simulink model "BetaMacs"  (R2023a)
settings: Solver=ode4  StartTime=0.0  StopTime=tsim  FixedStep=baseRate  RelTol=1e-6  AbsTol=1e-6
undefined symbols (not defined in the file): a1, a2, a3, b0, b1, b2, b3, baseRate, DiscIntNeverNeededParam, drop_states_ARM, drop_states_BLACK, drop_states_BLUE, drop_states_RED, F_Black_X_nominal, F_Black_Y_nominal, F_Blue_X_nominal, F_Blue_Y_nominal, F_red_X_nominal, F_red_Y_nominal, F_thrusters_BLACK, F_thrusters_BLUE, F_thrusters_RED, Gamma1_el, Gamma1_sh, Gamma1_wr, Gamma2_el, Gamma2_sh, Gamma2_wr, Gamma3_el, Gamma3_sh, Gamma3_wr, Gamma4_el, Gamma4_sh, Gamma4_wr, Gamma5_el, Gamma5_sh, Gamma5_wr, Gamma6_el, Gamma6_sh, Gamma6_wr, home_states_BLACK, home_states_BLUE, home_states_RED, IBLACK, IBLUE, IDIST, IEE, init_states_BLACK, init_states_BLUE, init_states_RED, IPROX, IRED, Kd_elarm, Kd_sharm, Kd_tb, Kd_tblue, Kd_tr, Kd_wrarm, Kd_xb, Kd_xblue ... (+48)
libraries: nvidiaSharedBlocks x9, MainLibrary x4, dspsigops x4, simulink x1
(part 2 of 11)

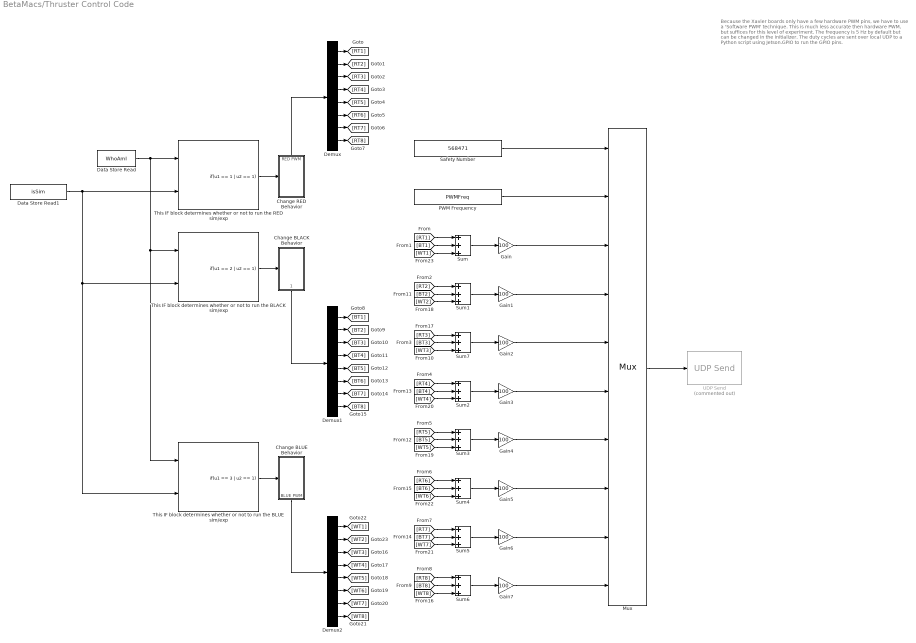
== system BetaMacs/Thruster Control Code ==
  note: Because the Xavier boards only have a few hardware PWM pins, we have to use a 'Software PWM' technique. This is much less accurate then hardware PWM, but suffices for this level of experiment.
      |
      | The frequency is 5 Hz by default but can be changed in the initializer. The duty cycles are sent over local UDP to a Python script using Jetson.GPIO to run the GPIO pins.
  Change BLACK Behavior : Subsystem  TreatAsAtomicUnit=on
  Change BLUE Behavior : Subsystem  TreatAsAtomicUnit=on
  Change RED Behavior : Subsystem  TreatAsAtomicUnit=on
  Data Store Read : DataStoreRead  DataStoreName=WhoAmI  IndexOptions=Index vector (dialog)  Indices=1  OutputSizes=1
  Data Store Read1 : DataStoreRead  DataStoreName=isSim  IndexOptions=Index vector (dialog)  Indices=1  OutputSizes=1
  Demux : Demux  Outputs=8
  Demux1 : Demux  Outputs=8
  Demux2 : Demux  Outputs=8
  Gain{,1..7} (8 alike) : Gain  Gain=100
  Mux : Mux  Inputs=10
  PWM Frequency : Constant  Value=PWMFreq
  Safety Number : Constant  Value=568471
  Sum{,1..7} (8 alike) : Sum  Inputs=+++
  This IF block determines whether or not to run the BLACK sim/exp : If  NumInputs=2  IfExpression=u1 == 2 | u2 == 1  ShowElse=off
  This IF block determines whether or not to run the BLUE sim/exp : If  NumInputs=2  IfExpression=u1 == 3 | u2 == 1  ShowElse=off
  "This IF block determines whether or not to run the RED sim/exp " : If  NumInputs=2  IfExpression=u1 == 1 | u2 == 1  ShowElse=off
  UDP Send : nvidiaSharedBlocks/UDP Send  Commented=on  remoteURL='127.0.0.1'  remotePort=48291  localURL='0.0.0.0'  localPortSource=Automatically determine  localPort=-1  sampletime=-1  blockPlatform=NVIDIA  separateLengthPort=0
      settings: LibrarySourceBlock=nvidiaNetworklib/UDP Send
  wires:
  Data Store Read1/1 -> This IF block determines whether or not to run the BLACK sim/exp/2, This IF block determines whether or not to run the BLUE sim/exp/2, "This IF block determines whether or not to run the RED sim/exp "/2
  "This IF block determines whether or not to run the RED sim/exp "/1 -> Change RED Behavior/Action
  This IF block determines whether or not to run the BLACK sim/exp/1 -> Change BLACK Behavior/Action
  Change RED Behavior/1(RED PWM) -> Demux/1
  Demux/1 -> [RT1]
  Demux/2 -> [RT2]
  Demux/3 -> [RT3]
  Demux/4 -> [RT4]
  Demux/5 -> [RT5]
  Demux/6 -> [RT6]
  Demux/7 -> [RT7]
  Demux/8 -> [RT8]
  Demux1/5 -> [BT5]
  Demux1/4 -> [BT4]
  Demux1/1 -> [BT1]
  Demux1/8 -> [BT8]
  Demux1/2 -> [BT2]
  Demux1/7 -> [BT7]
  Demux1/6 -> [BT6]
  Demux1/3 -> [BT3]
  Change BLACK Behavior/1(BLACK PWM) -> Demux1/1
  [RT1] -> Sum/1
  [BT1] -> Sum/2
  [RT2] -> Sum1/1
  [RT4] -> Sum2/1
  [RT5] -> Sum3/1
  [RT6] -> Sum4/1
  [RT7] -> Sum5/1
  [RT8] -> Sum6/1
  [BT8] -> Sum6/2
  [BT2] -> Sum1/2
  [BT5] -> Sum3/2
  [BT4] -> Sum2/2
  [BT7] -> Sum5/2
  [BT6] -> Sum4/2
  Sum/1 -> Gain/1
  Sum1/1 -> Gain1/1
  Data Store Read/1 -> This IF block determines whether or not to run the BLUE sim/exp/1, This IF block determines whether or not to run the BLACK sim/exp/1, "This IF block determines whether or not to run the RED sim/exp "/1
  This IF block determines whether or not to run the BLUE sim/exp/1 -> Change BLUE Behavior/Action
  Demux2/5 -> [WT5]
  Demux2/8 -> [WT8]
  Demux2/7 -> [WT7]
  Demux2/2 -> [WT2]
  Change BLUE Behavior/1(BLUE PWM) -> Demux2/1
  Demux2/1 -> [WT1]
  Demux2/4 -> [WT4]
  Demux2/3 -> [WT3]
  Demux2/6 -> [WT6]
  [WT8] -> Sum6/3
  [WT2] -> Sum1/3
  [WT5] -> Sum3/3
  [WT4] -> Sum2/3
  [WT7] -> Sum5/3
  [WT6] -> Sum4/3
  [WT1] -> Sum/3
  [BT3] -> Sum7/2
  [WT3] -> Sum7/3
  [RT3] -> Sum7/1
  Sum7/1 -> Gain2/1
  Sum2/1 -> Gain3/1
  Sum3/1 -> Gain4/1
  Sum5/1 -> Gain6/1
  Sum6/1 -> Gain7/1
  Sum4/1 -> Gain5/1
  Gain7/1 -> Mux/10
  Gain6/1 -> Mux/9
  Gain5/1 -> Mux/8
  Gain4/1 -> Mux/7
  Gain3/1 -> Mux/6
  Gain2/1 -> Mux/5
  Gain1/1 -> Mux/4
  Gain/1 -> Mux/3
  PWM Frequency/1 -> Mux/2
  Safety Number/1 -> Mux/1
  Mux/1 -> UDP Send/1

== system BetaMacs/Check Connection/Change BLACK Behavior ==
  Action Port : ActionPort  ActionPortLabel=if(u1 == 2 & u2 == 0)
  Constant1 : Constant  OutDataTypeStr=int32
  UDP Send : nvidiaSharedBlocks/UDP Send  remoteURL='255.255.255.255'  remotePort=33002  localURL='0.0.0.0'  localPortSource=Automatically determine  localPort=-1  sampletime=-1  blockPlatform=NVIDIA  separateLengthPort=0
      settings: LibrarySourceBlock=nvidiaNetworklib/UDP Send
  wires:
  Constant1/1 -> UDP Send/1

== system BetaMacs/Check Connection/Change BLUE Behavior ==
  Action Port : ActionPort  ActionPortLabel=if(u1 == 3 & u2 == 0)
  Constant1 : Constant  OutDataTypeStr=int32
  UDP Send : nvidiaSharedBlocks/UDP Send  remoteURL='255.255.255.255'  remotePort=33003  localURL='0.0.0.0'  localPortSource=Automatically determine  localPort=-1  sampletime=-1  blockPlatform=NVIDIA  separateLengthPort=0
      settings: LibrarySourceBlock=nvidiaNetworklib/UDP Send
  wires:
  Constant1/1 -> UDP Send/1

== system BetaMacs/Check Connection/Change RED Behavior ==
  Action Port : ActionPort  ActionPortLabel=if(u1 == 1 & u2 == 0)
  Constant1 : Constant  OutDataTypeStr=int32
  Terminator3 : Terminator
  UDP Send : nvidiaSharedBlocks/UDP Send  remoteURL='255.255.255.255'  remotePort=33001  localURL='0.0.0.0'  localPortSource=Automatically determine  localPort=-1  sampletime=-1  blockPlatform=NVIDIA  separateLengthPort=0
      settings: LibrarySourceBlock=nvidiaNetworklib/UDP Send
  wires:
  Constant1/1 -> UDP Send/1
  ? -> Terminator3/1

== system BetaMacs/Float Code/Enable Pucks ==
  Action Port : ActionPort  ActionPortLabel=if(u1 == 0)
  Data Store Read1 : DataStoreRead  DataStoreName=Float_State  IndexOptions=Index vector (dialog)  Indices=1  OutputSizes=1
  Set Pin 428 (Pucks) to HIGH : MATLABSystem  System=GPIO_Write  gpioPin=428  pinDirection=1
      mask Type: GPIO_Write
      mask Display:
      | disp('GPIO_Write');
      | port_label('input',1,'u');
  wires:
  Data Store Read1/1 -> Set Pin 428 (Pucks) to HIGH/1

== system BetaMacs/Manipulator Encoder Data/Change RED Behavior ==
  Action Port : ActionPort  ActionPortLabel=if(u1 == 1 & u2 == 0)
  Data Store Write : DataStoreWrite  DataStoreName=RED_Rz_Shoulder  IndexOptions=Index vector (dialog)  Indices=1  OutputSizes=1
  Data Store Write1 : DataStoreWrite  DataStoreName=RED_Rz_Elbow  IndexOptions=Index vector (dialog)  Indices=1  OutputSizes=1
  Data Store Write2 : DataStoreWrite  DataStoreName=RED_Rz_Wrist  IndexOptions=Index vector (dialog)  Indices=1  OutputSizes=1
  Data Store Write3 : DataStoreWrite  DataStoreName=RED_RzD_Shoulder  IndexOptions=Index vector (dialog)  Indices=1  OutputSizes=1
  Data Store Write4 : DataStoreWrite  DataStoreName=RED_RzD_Elbow  IndexOptions=Index vector (dialog)  Indices=1  OutputSizes=1
  Data Store Write5 : DataStoreWrite  DataStoreName=RED_RzD_Wrist  IndexOptions=Index vector (dialog)  Indices=1  OutputSizes=1
  Delay : Delay  DelayLength=1
  Delay1 : Delay  DelayLength=1
  Delay2 : Delay  DelayLength=1
  Read Joint Positions using Dynamixel Encoders : MainLibrary/Dynamixel Functions/Read Joint Positions using  Dynamixel Encoders  SampleTime=baseRate
  wires:
  Delay/1 -> Read Joint Positions using Dynamixel Encoders/1
  Read Joint Positions using Dynamixel Encoders/5 -> Data Store Write4/1
  Read Joint Positions using Dynamixel Encoders/6 -> Data Store Write5/1
  Delay1/1 -> Read Joint Positions using Dynamixel Encoders/2
  Read Joint Positions using Dynamixel Encoders/2 -> Delay1/1, Data Store Write1/1
  Delay2/1 -> Read Joint Positions using Dynamixel Encoders/3
  Read Joint Positions using Dynamixel Encoders/1 -> Delay/1, Data Store Write/1
  Read Joint Positions using Dynamixel Encoders/3 -> Delay2/1, Data Store Write2/1
  Read Joint Positions using Dynamixel Encoders/4 -> Data Store Write3/1

== system BetaMacs/Phase #0: Synchronization/Change BLACK Behavior ==
  note: Before getting good data, the platforms must NOT be floating. So, float is set to be "off".
  note: For the initialization phase, we do not want any thrust. Thus, all commanded forces are zero.
  Action Port : ActionPort  ActionPortLabel=if(u1 == 2 | u2 == 1)
  BLACK_Fx : DataStoreWrite  DataStoreName=BLACK_Fx  IndexOptions=Index vector (dialog)  Indices=1  OutputSizes=1
  BLACK_Fy : DataStoreWrite  DataStoreName=BLACK_Fy  IndexOptions=Index vector (dialog)  Indices=1  OutputSizes=1
  BLACK_Tz : DataStoreWrite  DataStoreName=BLACK_Tz  IndexOptions=Index vector (dialog)  Indices=1  OutputSizes=1
  Constant3 : Constant  Value=0
  Constant4 : Constant  Value=0
  Constant5 : Constant  Value=0
  Data Store Write4 : DataStoreWrite  DataStoreName=Float_State  IndexOptions=Index vector (dialog)  Indices=1  OutputSizes=1
  Puck State : Constant  Value=0
  wires:
  Constant3/1 -> BLACK_Fx/1
  Constant5/1 -> BLACK_Tz/1
  Constant4/1 -> BLACK_Fy/1
  Puck State/1 -> Data Store Write4/1

== system BetaMacs/Phase #0: Synchronization/Change BLUE Behavior ==
  note: Before getting good data, the platforms must NOT be floating. So, float is set to be "off".
  note: For the initialization phase, we do not want any thrust. Thus, all commanded forces are zero.
  Action Port : ActionPort  ActionPortLabel=if(u1 == 3 | u2 == 1)
  BLUE_Fx : DataStoreWrite  DataStoreName=BLUE_Fx  IndexOptions=Index vector (dialog)  Indices=1  OutputSizes=1
  BLUE_Fy : DataStoreWrite  DataStoreName=BLUE_Fy  IndexOptions=Index vector (dialog)  Indices=1  OutputSizes=1
  BLUE_Tz : DataStoreWrite  DataStoreName=BLUE_Tz  IndexOptions=Index vector (dialog)  Indices=1  OutputSizes=1
  Constant3 : Constant  Value=0
  Constant4 : Constant  Value=0
  Constant5 : Constant  Value=0
  Data Store Write4 : DataStoreWrite  DataStoreName=Float_State  IndexOptions=Index vector (dialog)  Indices=1  OutputSizes=1
  Puck State : Constant  Value=0
  wires:
  Constant3/1 -> BLUE_Fx/1
  Constant5/1 -> BLUE_Tz/1
  Constant4/1 -> BLUE_Fy/1
  Puck State/1 -> Data Store Write4/1

== system BetaMacs/Phase #0: Synchronization/Change RED Behavior ==
  note: For the initialization phase, we do not want any thrust or movement from the robotic arm. Thus, all commanded forces are zero.
  note: Before getting good data, the platforms must NOT be floating. So, float is set to be "off".
  Action Port : ActionPort  ActionPortLabel=if(u1 == 1 | u2 == 1)
  Constant{,1..4} (5 alike) : Constant  Value=0
  Data Store Write1 : DataStoreWrite  DataStoreName=RED_ARM_Control_Mode  IndexOptions=Index vector (dialog)  Indices=1  OutputSizes=1
  Data Store Write4 : DataStoreWrite  DataStoreName=Float_State  IndexOptions=Index vector (dialog)  Indices=1  OutputSizes=1
  Puck State : Constant  Value=0
  RED_Fx : DataStoreWrite  DataStoreName=RED_Fx  IndexOptions=Index vector (dialog)  Indices=1  OutputSizes=1
  RED_Fy : DataStoreWrite  DataStoreName=RED_Fy  IndexOptions=Index vector (dialog)  Indices=1  OutputSizes=1
  RED_Tz : DataStoreWrite  DataStoreName=RED_Tz  IndexOptions=Index vector (dialog)  Indices=1  OutputSizes=1
  RED_Tz_RW : DataStoreWrite  DataStoreName=RED_Tz_RW  IndexOptions=Index vector (dialog)  Indices=1  OutputSizes=1
  wires:
  Constant1/1 -> RED_Fy/1
  Constant2/1 -> RED_Tz/1
  Constant/1 -> RED_Fx/1
  Constant3/1 -> RED_Tz_RW/1
  Puck State/1 -> Data Store Write4/1
  Constant4/1 -> Data Store Write1/1

== system BetaMacs/Phase #1: Start Floating /Change BLACK Behavior ==
  note: For the float phase, we do not want any thrust. Thus, all commanded forces are zero.
  note: Now that good data is available, the platform can start to float.
  Action Port : ActionPort  ActionPortLabel=if(u1 == 2 | u2 == 1)
  BLACK_Fx : DataStoreWrite  DataStoreName=BLACK_Fx  IndexOptions=Index vector (dialog)  Indices=1  OutputSizes=1
  BLACK_Fy : DataStoreWrite  DataStoreName=BLACK_Fy  IndexOptions=Index vector (dialog)  Indices=1  OutputSizes=1
  BLACK_Tz : DataStoreWrite  DataStoreName=BLACK_Tz  IndexOptions=Index vector (dialog)  Indices=1  OutputSizes=1
  Constant3 : Constant  Value=0
  Constant4 : Constant  Value=0
  Constant5 : Constant  Value=0
  Data Store Write4 : DataStoreWrite  DataStoreName=Float_State  IndexOptions=Index vector (dialog)  Indices=1  OutputSizes=1
  Puck State : Constant
  wires:
  Constant3/1 -> BLACK_Fx/1
  Constant5/1 -> BLACK_Tz/1
  Constant4/1 -> BLACK_Fy/1
  Puck State/1 -> Data Store Write4/1

== system BetaMacs/Phase #1: Start Floating /Change BLUE Behavior ==
  note: Before getting good data, the platforms must NOT be floating. So, float is set to be "off".
  note: For the initialization phase, we do not want any thrust. Thus, all commanded forces are zero.
  Action Port : ActionPort  ActionPortLabel=if(u1 == 3 | u2 == 1)
  BLUE_Fx : DataStoreWrite  DataStoreName=BLUE_Fx  IndexOptions=Index vector (dialog)  Indices=1  OutputSizes=1
  BLUE_Fy : DataStoreWrite  DataStoreName=BLUE_Fy  IndexOptions=Index vector (dialog)  Indices=1  OutputSizes=1
  BLUE_Tz : DataStoreWrite  DataStoreName=BLUE_Tz  IndexOptions=Index vector (dialog)  Indices=1  OutputSizes=1
  Constant3 : Constant  Value=0
  Constant4 : Constant  Value=0
  Constant5 : Constant  Value=0
  Data Store Write4 : DataStoreWrite  DataStoreName=Float_State  IndexOptions=Index vector (dialog)  Indices=1  OutputSizes=1
  Puck State : Constant
  wires:
  Constant3/1 -> BLUE_Fx/1
  Constant5/1 -> BLUE_Tz/1
  Constant4/1 -> BLUE_Fy/1
  Puck State/1 -> Data Store Write4/1

== system BetaMacs/Phase #1: Start Floating /Change RED Behavior ==
  note: Now that good data is available, the platforms can start to float.
  note: For the float phase, we do not want any thrust or movement from the robotic arm. Thus, all commanded forces are zero.
  Action Port : ActionPort  ActionPortLabel=if(u1 == 1 | u2 == 1)
  Constant{,1..4} (5 alike) : Constant  Value=0
  Data Store Write1 : DataStoreWrite  DataStoreName=RED_ARM_Control_Mode  IndexOptions=Index vector (dialog)  Indices=1  OutputSizes=1
  Data Store Write4 : DataStoreWrite  DataStoreName=Float_State  IndexOptions=Index vector (dialog)  Indices=1  OutputSizes=1
  Puck State : Constant
  RED_Fx : DataStoreWrite  DataStoreName=RED_Fx  IndexOptions=Index vector (dialog)  Indices=1  OutputSizes=1
  RED_Fy : DataStoreWrite  DataStoreName=RED_Fy  IndexOptions=Index vector (dialog)  Indices=1  OutputSizes=1
  RED_Tz : DataStoreWrite  DataStoreName=RED_Tz  IndexOptions=Index vector (dialog)  Indices=1  OutputSizes=1
  RED_Tz_RW : DataStoreWrite  DataStoreName=RED_Tz_RW  IndexOptions=Index vector (dialog)  Indices=1  OutputSizes=1
  wires:
  Constant/1 -> RED_Fx/1
  Constant3/1 -> RED_Tz_RW/1
  Constant2/1 -> RED_Tz/1
  Constant1/1 -> RED_Fy/1
  Puck State/1 -> Data Store Write4/1
  Constant4/1 -> Data Store Write1/1

== system BetaMacs/Phase #2: Initial Position/Change BLACK Behavior ==
  note: Additional Blocks
  note: PD Control Law - BLACK
  note: Additional blocks are stored here.
  note: A simple PD control law is used here to command the platform to it's initial position, as defined in the initializer.
  Action Port : ActionPort  ActionPortLabel=if(u1 == 2 | u2 == 1)
  BLACK_Fx : DataStoreWrite  DataStoreName=BLACK_Fx  IndexOptions=Index vector (dialog)  Indices=1  OutputSizes=1
  BLACK_Fy : DataStoreWrite  DataStoreName=BLACK_Fy  IndexOptions=Index vector (dialog)  Indices=1  OutputSizes=1
  BLACK_Px : DataStoreRead  DataStoreName=BLACK_Px  IndexOptions=Index vector (dialog)  Indices=1  OutputSizes=1
  "BLACK_Py " : DataStoreRead  DataStoreName=BLACK_Py  IndexOptions=Index vector (dialog)  Indices=1  OutputSizes=1
  BLACK_Rz : DataStoreRead  DataStoreName=BLACK_Rz  IndexOptions=Index vector (dialog)  Indices=1  OutputSizes=1
  BLACK_Tz : DataStoreWrite  DataStoreName=BLACK_Tz  IndexOptions=Index vector (dialog)  Indices=1  OutputSizes=1
  Custom Discrete PD (Attitude) : Subsystem
  Custom Discrete PD (X-Position) : Subsystem
  Custom Discrete PD (Y-Position) : Subsystem
  Data Store Write3 : DataStoreWrite  DataStoreName=Float_State  IndexOptions=Index vector (dialog)  Indices=1  OutputSizes=1
  Desired Attitude (BLACK) : Constant  Value=init_states_BLACK(3)  SampleTime=-1
  Desired Px (BLACK) : Constant  Value=init_states_BLACK(1)  SampleTime=-1
  Desired Py (BLACK) : Constant  Value=init_states_BLACK(2)  SampleTime=-1
  Hough Control : Subsystem
  Puck State : Constant
  Subtract : Sum  Inputs=+-
  Subtract1 : Sum  Inputs=+-
  wires:
  Custom Discrete PD (Y-Position)/1(Fy) -> BLACK_Fy/1
  Hough Control/1(Err) -> Custom Discrete PD (Attitude)/1(ez)
  BLACK_Px/1 -> Subtract/2
  Subtract1/1 -> Custom Discrete PD (Y-Position)/1(ey)
  Custom Discrete PD (Attitude)/1(Tz) -> BLACK_Tz/1
  "BLACK_Py "/1 -> Subtract1/2
  Subtract/1 -> Custom Discrete PD (X-Position)/1(ex)
  Custom Discrete PD (X-Position)/1(Fx) -> BLACK_Fx/1
  Desired Px (BLACK)/1 -> Subtract/1
  Desired Py (BLACK)/1 -> Subtract1/1
  Desired Attitude (BLACK)/1 -> Hough Control/1(Ref)
  BLACK_Rz/1 -> Hough Control/2(Act)
  Puck State/1 -> Data Store Write3/1

== system BetaMacs/Phase #2: Initial Position/Change BLUE Behavior ==
  note: PD Control Law - BLUE
  note: Additional blocks are stored here.
  note: A simple PD control law is used here to command the platform to it's initial position, as defined in the initializer.
  note: Additional Blocks
  Action Port : ActionPort  ActionPortLabel=if(u1 == 3 | u2 == 1)
  BLUE_Fx : DataStoreWrite  DataStoreName=BLUE_Fx  IndexOptions=Index vector (dialog)  Indices=1  OutputSizes=1
  BLUE_Fy : DataStoreWrite  DataStoreName=BLUE_Fy  IndexOptions=Index vector (dialog)  Indices=1  OutputSizes=1
  BLUE_Px : DataStoreRead  DataStoreName=BLUE_Px  IndexOptions=Index vector (dialog)  Indices=1  OutputSizes=1
  "BLUE_Py " : DataStoreRead  DataStoreName=BLUE_Py  IndexOptions=Index vector (dialog)  Indices=1  OutputSizes=1
  BLUE_Rz : DataStoreRead  DataStoreName=BLUE_Rz  IndexOptions=Index vector (dialog)  Indices=1  OutputSizes=1
  BLUE_Tz : DataStoreWrite  DataStoreName=BLUE_Tz  IndexOptions=Index vector (dialog)  Indices=1  OutputSizes=1
  Custom Discrete PD (Attitude) : Subsystem
  Custom Discrete PD (X-Position) : Subsystem
  Custom Discrete PD (Y-Position) : Subsystem
  Data Store Write3 : DataStoreWrite  DataStoreName=Float_State  IndexOptions=Index vector (dialog)  Indices=1  OutputSizes=1
  Desired Attitude (BLUE) : Constant  Value=init_states_BLUE(3)  SampleTime=-1
  Desired Px (BLUE) : Constant  Value=init_states_BLUE(1)  SampleTime=-1
  Desired Py (BLUE) : Constant  Value=init_states_BLUE(2)  SampleTime=-1
  Hough Control : Subsystem
  Puck State : Constant
  Subtract : Sum  Inputs=+-
  Subtract1 : Sum  Inputs=+-
  wires:
  Desired Attitude (BLUE)/1 -> Hough Control/1(Ref)
  BLUE_Rz/1 -> Hough Control/2(Act)
  Puck State/1 -> Data Store Write3/1
  Subtract/1 -> Custom Discrete PD (X-Position)/1(ex)
  Hough Control/1(Err) -> Custom Discrete PD (Attitude)/1(ez)
  Custom Discrete PD (X-Position)/1(Fx) -> BLUE_Fx/1
  Desired Py (BLUE)/1 -> Subtract1/1
  BLUE_Px/1 -> Subtract/2
  Subtract1/1 -> Custom Discrete PD (Y-Position)/1(ey)
  Desired Px (BLUE)/1 -> Subtract/1
  "BLUE_Py "/1 -> Subtract1/2
  Custom Discrete PD (Y-Position)/1(Fy) -> BLUE_Fy/1
  Custom Discrete PD (Attitude)/1(Tz) -> BLUE_Tz/1

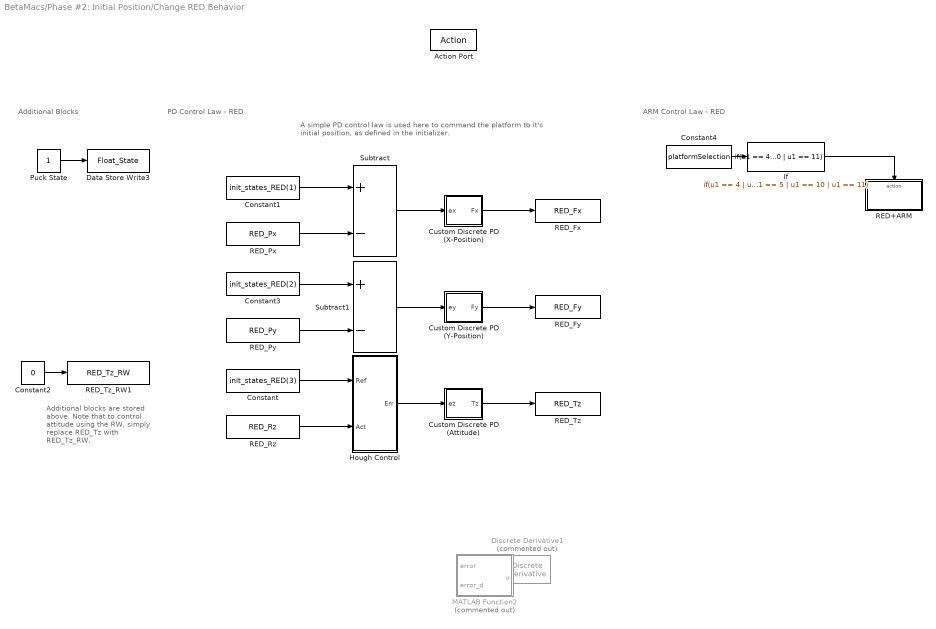
== system BetaMacs/Phase #2: Initial Position/Change RED Behavior ==
  note: PD Control Law - RED
  note: Additional Blocks
  note: Additional blocks are stored above. Note that to control attitude using the RW, simply replace RED_Tz with RED_Tz_RW.
  note: A simple PD control law is used here to command the platform to it's initial position, as defined in the initializer.
  note: ARM Control Law - RED
  Action Port : ActionPort  ActionPortLabel=if(u1 == 1 | u2 == 1)
  Constant : Constant  Value=init_states_RED(3)
  Constant1 : Constant  Value=init_states_RED(1)
  Constant2 : Constant  Value=0
  Constant3 : Constant  Value=init_states_RED(2)
  Constant4 : Constant  Value=platformSelection
  Custom Discrete PD (Attitude) : Subsystem
  Custom Discrete PD (X-Position) : Subsystem
  Custom Discrete PD (Y-Position) : Subsystem
  Data Store Write3 : DataStoreWrite  DataStoreName=Float_State  IndexOptions=Index vector (dialog)  Indices=1  OutputSizes=1
  Discrete Derivative1 : simulink/Discrete/Discrete Derivative  Commented=on  gainval=1.0  ICPrevScaledInput=0.0  OutMin=[]  OutMax=[]  OutDataType=fixdt(1, 16)  OutScaling=2^-10  DoSatur=off
  Hough Control : Subsystem
  If : If  IfExpression=u1 == 4 | u1 == 5 | u1 == 10 | u1 == 11  ShowElse=off
  MATLAB Function2 : MATLAB Function  Commented=on  TreatAsAtomicUnit=on
  Puck State : Constant
  RED+ARM : Subsystem  TreatAsAtomicUnit=on
  RED_Fx : DataStoreWrite  DataStoreName=RED_Fx  IndexOptions=Index vector (dialog)  Indices=1  OutputSizes=1
  RED_Fy : DataStoreWrite  DataStoreName=RED_Fy  IndexOptions=Index vector (dialog)  Indices=1  OutputSizes=1
  RED_Px : DataStoreRead  DataStoreName=RED_Px  IndexOptions=Index vector (dialog)  Indices=1  OutputSizes=1
  "RED_Py " : DataStoreRead  DataStoreName=RED_Py  IndexOptions=Index vector (dialog)  Indices=1  OutputSizes=1
  RED_Rz : DataStoreRead  DataStoreName=RED_Rz  IndexOptions=Index vector (dialog)  Indices=1  OutputSizes=1
  RED_Tz : DataStoreWrite  DataStoreName=RED_Tz  IndexOptions=Index vector (dialog)  Indices=1  OutputSizes=1
  RED_Tz_RW1 : DataStoreWrite  DataStoreName=RED_Tz_RW  IndexOptions=Index vector (dialog)  Indices=1  OutputSizes=1
  Subtract : Sum  Inputs=+-
  Subtract1 : Sum  Inputs=+-
  wires:
  Constant2/1 -> RED_Tz_RW1/1
  RED_Rz/1 -> Hough Control/2(Act)
  RED_Px/1 -> Subtract/2
  "RED_Py "/1 -> Subtract1/2
  Constant1/1 -> Subtract/1
  Constant3/1 -> Subtract1/1
  Constant/1 -> Hough Control/1(Ref)
  Puck State/1 -> Data Store Write3/1
  Constant4/1 -> If/1
  If/1 -> RED+ARM/Action
  Custom Discrete PD (X-Position)/1(Fx) -> RED_Fx/1
  Subtract/1 -> Custom Discrete PD (X-Position)/1(ex)
  Subtract1/1 -> Custom Discrete PD (Y-Position)/1(ey)
  Custom Discrete PD (Y-Position)/1(Fy) -> RED_Fy/1
  Custom Discrete PD (Attitude)/1(Tz) -> RED_Tz/1
  Hough Control/1(Err) -> Custom Discrete PD (Attitude)/1(ez)

== system BetaMacs/Phase #3: Experiment/Change BLACK Behavior ==
  note: For experiments, it is usually desirable to have various sub-phases. The sub-phases are defined in the initializer; note that in the template only three sub-phases are present, but more can be added.
  Action Port : ActionPort  ActionPortLabel=if(u1 == 2 | u2 == 1)
  Constant1 : Constant  Value=Phase3_SubPhase2_End  SampleTime=-1
  Constant2 : Constant  Value=Phase3_SubPhase3_End  SampleTime=-1
  Constant3 : Constant  Value=Phase3_SubPhase4_End  SampleTime=-1
  Constant4 : Constant  Value=Phase3_SubPhase1_End  SampleTime=-1
  Experiment Sub-Phases : If  NumInputs=5  IfExpression=u1 < u2  ElseIfExpressions=(u1 < u3 & u1 >= u2),(u1 < u4 & u1 >= u3), (u1 < u5 & u1 >= u4)  ShowElse=off
  Sub-Phase #1 : Subsystem  TreatAsAtomicUnit=on
  "Sub-Phase #2 " : Subsystem  TreatAsAtomicUnit=on
  "Sub-Phase #3 " : Subsystem  TreatAsAtomicUnit=on
  Sub-Phase #4 : Subsystem  TreatAsAtomicUnit=on
  Universal_Time : DataStoreRead  DataStoreName=Univ_Time  IndexOptions=Index vector (dialog)  Indices=1  OutputSizes=1
  wires:
  Experiment Sub-Phases/2 -> "Sub-Phase #2 "/Action
  Experiment Sub-Phases/1 -> Sub-Phase #1/Action
  Experiment Sub-Phases/3 -> "Sub-Phase #3 "/Action
  Constant1/1 -> Experiment Sub-Phases/3
  Constant2/1 -> Experiment Sub-Phases/4
  Constant4/1 -> Experiment Sub-Phases/2
  Universal_Time/1 -> Experiment Sub-Phases/1
  Constant3/1 -> Experiment Sub-Phases/5
  Experiment Sub-Phases/4 -> Sub-Phase #4/Action

== system BetaMacs/Phase #3: Experiment/Change BLUE Behavior ==
  Action Port : ActionPort  ActionPortLabel=if(u1 == 3 | u2 == 1)
  Constant1 : Constant  Value=Phase3_SubPhase2_End  SampleTime=-1
  Constant2 : Constant  Value=Phase3_SubPhase3_End  SampleTime=-1
  Constant3 : Constant  Value=Phase3_SubPhase4_End  SampleTime=-1
  Constant4 : Constant  Value=Phase3_SubPhase1_End  SampleTime=-1
  Experiment Sub-Phases : If  NumInputs=5  IfExpression=u1 < u2  ElseIfExpressions=(u1 < u3 & u1 >= u2),(u1 < u4 & u1 >= u3), (u1 < u5 & u1 >= u4)  ShowElse=off
  Sub-Phase #1 : Subsystem  TreatAsAtomicUnit=on
  "Sub-Phase #2 " : Subsystem  TreatAsAtomicUnit=on
  "Sub-Phase #3 " : Subsystem  TreatAsAtomicUnit=on
  Sub-Phase #4 : Subsystem  TreatAsAtomicUnit=on
  Universal_Time : DataStoreRead  DataStoreName=Univ_Time  IndexOptions=Index vector (dialog)  Indices=1  OutputSizes=1
  wires:
  Constant3/1 -> Experiment Sub-Phases/5
  Experiment Sub-Phases/4 -> Sub-Phase #4/Action
  Universal_Time/1 -> Experiment Sub-Phases/1
  Experiment Sub-Phases/1 -> Sub-Phase #1/Action
  Constant2/1 -> Experiment Sub-Phases/4
  Constant4/1 -> Experiment Sub-Phases/2
  Constant1/1 -> Experiment Sub-Phases/3
  Experiment Sub-Phases/3 -> "Sub-Phase #3 "/Action
  Experiment Sub-Phases/2 -> "Sub-Phase #2 "/Action

== system BetaMacs/Phase #3: Experiment/Change RED Behavior ==
  note: For experiments, it is usually desirable to have various sub-phases. The sub-phases are defined in the initializer; note that in the template only three sub-phases are present, but more can be added.
  Action Port : ActionPort  ActionPortLabel=if(u1 == 1 | u2 == 1)
  Constant1 : Constant  Value=Phase3_SubPhase2_End  SampleTime=-1
  Constant2 : Constant  Value=Phase3_SubPhase3_End  SampleTime=-1
  Constant3 : Constant  Value=Phase3_SubPhase4_End  SampleTime=-1
  Constant4 : Constant  Value=Phase3_SubPhase1_End  SampleTime=-1
  Experiment Sub-Phases : If  NumInputs=5  IfExpression=u1 < u2  ElseIfExpressions=(u1 < u3 & u1 >= u2),(u1 < u4 & u1 >= u3), (u1 < u5 & u1 >= u4)  ShowElse=off
  Sub-Phase #1 : Subsystem  TreatAsAtomicUnit=on
  "Sub-Phase #2 " : Subsystem  TreatAsAtomicUnit=on
  "Sub-Phase #3 " : Subsystem  TreatAsAtomicUnit=on
  Sub-Phase #4 : Subsystem  TreatAsAtomicUnit=on
  Universal_Time : DataStoreRead  DataStoreName=Univ_Time  IndexOptions=Index vector (dialog)  Indices=1  OutputSizes=1
  wires:
  Experiment Sub-Phases/1 -> Sub-Phase #1/Action
  Experiment Sub-Phases/2 -> "Sub-Phase #2 "/Action
  Universal_Time/1 -> Experiment Sub-Phases/1
  Experiment Sub-Phases/3 -> "Sub-Phase #3 "/Action
  Constant4/1 -> Experiment Sub-Phases/2
  Constant1/1 -> Experiment Sub-Phases/3
  Constant2/1 -> Experiment Sub-Phases/4
  Constant3/1 -> Experiment Sub-Phases/5
  Experiment Sub-Phases/4 -> Sub-Phase #4/Action

== system BetaMacs/Phase #4: Return Home/Change BLACK Behavior ==
  note: Additional Blocks
  note: PD Control Law - BLACK
  note: Additional blocks are stored here.
  note: A simple PD control law is used here to command the platform to it's initial position, as defined in the initializer.
  Action Port : ActionPort  ActionPortLabel=if(u1 == 2 | u2 == 1)
  BLACK_Fx : DataStoreWrite  DataStoreName=BLACK_Fx  IndexOptions=Index vector (dialog)  Indices=1  OutputSizes=1
  BLACK_Fy : DataStoreWrite  DataStoreName=BLACK_Fy  IndexOptions=Index vector (dialog)  Indices=1  OutputSizes=1
  BLACK_Px : DataStoreRead  DataStoreName=BLACK_Px  IndexOptions=Index vector (dialog)  Indices=1  OutputSizes=1
  "BLACK_Py " : DataStoreRead  DataStoreName=BLACK_Py  IndexOptions=Index vector (dialog)  Indices=1  OutputSizes=1
  BLACK_Rz : DataStoreRead  DataStoreName=BLACK_Rz  IndexOptions=Index vector (dialog)  Indices=1  OutputSizes=1
  BLACK_Tz : DataStoreWrite  DataStoreName=BLACK_Tz  IndexOptions=Index vector (dialog)  Indices=1  OutputSizes=1
  Custom Discrete PD (Attitude) : Subsystem
  Custom Discrete PD (X-Position) : Subsystem
  Custom Discrete PD (Y-Position) : Subsystem
  Data Store Write3 : DataStoreWrite  DataStoreName=Float_State  IndexOptions=Index vector (dialog)  Indices=1  OutputSizes=1
  Desired Attitude (BLACK) : Constant  Value=home_states_BLACK(3)  SampleTime=-1
  Desired Px (BLACK) : Constant  Value=home_states_BLACK(1)  SampleTime=-1
  Desired Py (BLACK) : Constant  Value=home_states_BLACK(2)  SampleTime=-1
  Hough Control : Subsystem
  Puck State : Constant
  Subtract : Sum  Inputs=+-
  Subtract1 : Sum  Inputs=+-
  wires:
  Custom Discrete PD (Y-Position)/1(Fy) -> BLACK_Fy/1
  Desired Py (BLACK)/1 -> Subtract1/1
  Hough Control/1(Err) -> Custom Discrete PD (Attitude)/1(ez)
  BLACK_Px/1 -> Subtract/2
  Subtract1/1 -> Custom Discrete PD (Y-Position)/1(ey)
  Custom Discrete PD (Attitude)/1(Tz) -> BLACK_Tz/1
  Desired Attitude (BLACK)/1 -> Hough Control/1(Ref)
  "BLACK_Py "/1 -> Subtract1/2
  Subtract/1 -> Custom Discrete PD (X-Position)/1(ex)
  BLACK_Rz/1 -> Hough Control/2(Act)
  Desired Px (BLACK)/1 -> Subtract/1
  Custom Discrete PD (X-Position)/1(Fx) -> BLACK_Fx/1
  Puck State/1 -> Data Store Write3/1

== system BetaMacs/Phase #4: Return Home/Change BLUE Behavior ==
  note: PD Control Law - BLUE
  note: Additional blocks are stored here.
  note: A simple PD control law is used here to command the platform to it's initial position, as defined in the initializer.
  note: Additional Blocks
  Action Port : ActionPort  ActionPortLabel=if(u1 == 3 | u2 == 1)
  BLUE_Fx : DataStoreWrite  DataStoreName=BLUE_Fx  IndexOptions=Index vector (dialog)  Indices=1  OutputSizes=1
  BLUE_Fy : DataStoreWrite  DataStoreName=BLUE_Fy  IndexOptions=Index vector (dialog)  Indices=1  OutputSizes=1
  BLUE_Px : DataStoreRead  DataStoreName=BLUE_Px  IndexOptions=Index vector (dialog)  Indices=1  OutputSizes=1
  "BLUE_Py " : DataStoreRead  DataStoreName=BLUE_Py  IndexOptions=Index vector (dialog)  Indices=1  OutputSizes=1
  BLUE_Rz : DataStoreRead  DataStoreName=BLUE_Rz  IndexOptions=Index vector (dialog)  Indices=1  OutputSizes=1
  BLUE_Tz : DataStoreWrite  DataStoreName=BLUE_Tz  IndexOptions=Index vector (dialog)  Indices=1  OutputSizes=1
  Custom Discrete PD (Attitude) : Subsystem
  Custom Discrete PD (X-Position) : Subsystem
  Custom Discrete PD (Y-Position) : Subsystem
  Data Store Write3 : DataStoreWrite  DataStoreName=Float_State  IndexOptions=Index vector (dialog)  Indices=1  OutputSizes=1
  Desired Attitude (BLUE) : Constant  Value=home_states_BLUE(3)  SampleTime=-1
  Desired Px (BLUE) : Constant  Value=home_states_BLUE(1)  SampleTime=-1
  Desired Py (BLUE) : Constant  Value=home_states_BLUE(2)  SampleTime=-1
  Hough Control : Subsystem
  Puck State : Constant
  Subtract : Sum  Inputs=+-
  Subtract1 : Sum  Inputs=+-
  wires:
  Puck State/1 -> Data Store Write3/1
  Subtract/1 -> Custom Discrete PD (X-Position)/1(ex)
  Desired Py (BLUE)/1 -> Subtract1/1
  Custom Discrete PD (X-Position)/1(Fx) -> BLUE_Fx/1
  Desired Px (BLUE)/1 -> Subtract/1
  Subtract1/1 -> Custom Discrete PD (Y-Position)/1(ey)
  Hough Control/1(Err) -> Custom Discrete PD (Attitude)/1(ez)
  Desired Attitude (BLUE)/1 -> Hough Control/1(Ref)
  Custom Discrete PD (Attitude)/1(Tz) -> BLUE_Tz/1
  "BLUE_Py "/1 -> Subtract1/2
  Custom Discrete PD (Y-Position)/1(Fy) -> BLUE_Fy/1
  BLUE_Px/1 -> Subtract/2
  BLUE_Rz/1 -> Hough Control/2(Act)

== system BetaMacs/Phase #4: Return Home/Change RED Behavior ==
  note: PD Control Law - RED
  note: Additional Blocks
  note: Additional blocks are stored above. Note that to control attitude using the RW, simply replace RED_Tz with RED_Tz_RW.
  note: A simple PD control law is used here to command the platform to it's initial position, as defined in the initializer.
  note: ARM Control Law - RED
  Action Port : ActionPort  ActionPortLabel=if(u1 == 1 | u2 == 1)
  Constant2 : Constant  Value=0
  Constant4 : Constant  Value=platformSelection
  Custom Discrete PD (Attitude) : Subsystem
  Custom Discrete PD (X-Position) : Subsystem
  Custom Discrete PD (Y-Position) : Subsystem
  Data Store Write3 : DataStoreWrite  DataStoreName=Float_State  IndexOptions=Index vector (dialog)  Indices=1  OutputSizes=1
  Desired Px (RED) : Constant  Value=home_states_RED(1)  SampleTime=-1
  Desired Py (RED) : Constant  Value=home_states_RED(2)  SampleTime=-1
  Desired Rz (RED) : Constant  Value=home_states_RED(3)  SampleTime=-1
  Hough Control : Subsystem
  If : If  IfExpression=u1 == 4 | u1 == 5 | u1 == 10 | u1 == 11  ShowElse=off
  Puck State : Constant
  RED+ARM : Subsystem  TreatAsAtomicUnit=on
  RED_Fx : DataStoreWrite  DataStoreName=RED_Fx  IndexOptions=Index vector (dialog)  Indices=1  OutputSizes=1
  RED_Fy : DataStoreWrite  DataStoreName=RED_Fy  IndexOptions=Index vector (dialog)  Indices=1  OutputSizes=1
  RED_Px : DataStoreRead  DataStoreName=RED_Px  IndexOptions=Index vector (dialog)  Indices=1  OutputSizes=1
  "RED_Py " : DataStoreRead  DataStoreName=RED_Py  IndexOptions=Index vector (dialog)  Indices=1  OutputSizes=1
  RED_Rz : DataStoreRead  DataStoreName=RED_Rz  IndexOptions=Index vector (dialog)  Indices=1  OutputSizes=1
  RED_Tz : DataStoreWrite  DataStoreName=RED_Tz  IndexOptions=Index vector (dialog)  Indices=1  OutputSizes=1
  RED_Tz_RW1 : DataStoreWrite  DataStoreName=RED_Tz_RW  IndexOptions=Index vector (dialog)  Indices=1  OutputSizes=1
  Subtract : Sum  Inputs=+-
  Subtract1 : Sum  Inputs=+-
  wires:
  Constant2/1 -> RED_Tz_RW1/1
  Desired Px (RED)/1 -> Subtract/1
  Custom Discrete PD (Attitude)/1(Tz) -> RED_Tz/1
  Desired Rz (RED)/1 -> Hough Control/1(Ref)
  RED_Rz/1 -> Hough Control/2(Act)
  Desired Py (RED)/1 -> Subtract1/1
  Custom Discrete PD (X-Position)/1(Fx) -> RED_Fx/1
  Subtract/1 -> Custom Discrete PD (X-Position)/1(ex)
  Hough Control/1(Err) -> Custom Discrete PD (Attitude)/1(ez)
  Custom Discrete PD (Y-Position)/1(Fy) -> RED_Fy/1
  RED_Px/1 -> Subtract/2
  "RED_Py "/1 -> Subtract1/2
  Subtract1/1 -> Custom Discrete PD (Y-Position)/1(ey)
  Puck State/1 -> Data Store Write3/1
  Constant4/1 -> If/1
  If/1 -> RED+ARM/Action

== system BetaMacs/Phase #5: Hold Home/Change BLACK Behavior ==
  note: Additional Blocks
  note: PD Control Law - BLACK
  note: Additional blocks are stored here.
  note: A simple PD control law is used here to command the platform to it's initial position, as defined in the initializer.
  Action Port : ActionPort  ActionPortLabel=if(u1 == 2 | u2 == 1)
  BLACK_Fx : DataStoreWrite  DataStoreName=BLACK_Fx  IndexOptions=Index vector (dialog)  Indices=1  OutputSizes=1
  BLACK_Fy : DataStoreWrite  DataStoreName=BLACK_Fy  IndexOptions=Index vector (dialog)  Indices=1  OutputSizes=1
  BLACK_Px : DataStoreRead  DataStoreName=BLACK_Px  IndexOptions=Index vector (dialog)  Indices=1  OutputSizes=1
  "BLACK_Py " : DataStoreRead  DataStoreName=BLACK_Py  IndexOptions=Index vector (dialog)  Indices=1  OutputSizes=1
  BLACK_Rz : DataStoreRead  DataStoreName=BLACK_Rz  IndexOptions=Index vector (dialog)  Indices=1  OutputSizes=1
  BLACK_Tz : DataStoreWrite  DataStoreName=BLACK_Tz  IndexOptions=Index vector (dialog)  Indices=1  OutputSizes=1
  Custom Discrete PD (Attitude) : Subsystem
  Custom Discrete PD (X-Position) : Subsystem
  Custom Discrete PD (Y-Position) : Subsystem
  Data Store Write3 : DataStoreWrite  DataStoreName=Float_State  IndexOptions=Index vector (dialog)  Indices=1  OutputSizes=1
  Desired Attitude (BLACK) : Constant  Value=home_states_BLACK(3)  SampleTime=-1
  Desired Px (BLACK) : Constant  Value=home_states_BLACK(1)  SampleTime=-1
  Desired Py (BLACK) : Constant  Value=home_states_BLACK(2)  SampleTime=-1
  Hough Control : Subsystem
  Puck State : Constant
  Subtract : Sum  Inputs=+-
  Subtract1 : Sum  Inputs=+-
  wires:
  Custom Discrete PD (Y-Position)/1(Fy) -> BLACK_Fy/1
  Desired Py (BLACK)/1 -> Subtract1/1
  Hough Control/1(Err) -> Custom Discrete PD (Attitude)/1(ez)
  BLACK_Px/1 -> Subtract/2
  Subtract1/1 -> Custom Discrete PD (Y-Position)/1(ey)
  Custom Discrete PD (Attitude)/1(Tz) -> BLACK_Tz/1
  Desired Attitude (BLACK)/1 -> Hough Control/1(Ref)
  "BLACK_Py "/1 -> Subtract1/2
  Subtract/1 -> Custom Discrete PD (X-Position)/1(ex)
  BLACK_Rz/1 -> Hough Control/2(Act)
  Desired Px (BLACK)/1 -> Subtract/1
  Custom Discrete PD (X-Position)/1(Fx) -> BLACK_Fx/1
  Puck State/1 -> Data Store Write3/1

== system BetaMacs/Phase #5: Hold Home/Change BLUE Behavior ==
  note: PD Control Law - BLUE
  note: Additional blocks are stored here.
  note: A simple PD control law is used here to command the platform to it's initial position, as defined in the initializer.
  note: Additional Blocks
  Action Port : ActionPort  ActionPortLabel=if(u1 == 3 | u2 == 1)
  BLUE_Fx : DataStoreWrite  DataStoreName=BLUE_Fx  IndexOptions=Index vector (dialog)  Indices=1  OutputSizes=1
  BLUE_Fy : DataStoreWrite  DataStoreName=BLUE_Fy  IndexOptions=Index vector (dialog)  Indices=1  OutputSizes=1
  BLUE_Px : DataStoreRead  DataStoreName=BLUE_Px  IndexOptions=Index vector (dialog)  Indices=1  OutputSizes=1
  "BLUE_Py " : DataStoreRead  DataStoreName=BLUE_Py  IndexOptions=Index vector (dialog)  Indices=1  OutputSizes=1
  BLUE_Rz : DataStoreRead  DataStoreName=BLUE_Rz  IndexOptions=Index vector (dialog)  Indices=1  OutputSizes=1
  BLUE_Tz : DataStoreWrite  DataStoreName=BLUE_Tz  IndexOptions=Index vector (dialog)  Indices=1  OutputSizes=1
  Custom Discrete PD (Attitude) : Subsystem
  Custom Discrete PD (X-Position) : Subsystem
  Custom Discrete PD (Y-Position) : Subsystem
  Data Store Write3 : DataStoreWrite  DataStoreName=Float_State  IndexOptions=Index vector (dialog)  Indices=1  OutputSizes=1
  Desired Attitude (BLUE) : Constant  Value=home_states_BLUE(3)  SampleTime=-1
  Desired Px (BLUE) : Constant  Value=home_states_BLUE(1)  SampleTime=-1
  Desired Py (BLUE) : Constant  Value=home_states_BLUE(2)  SampleTime=-1
  Hough Control : Subsystem
  Puck State : Constant
  Subtract : Sum  Inputs=+-
  Subtract1 : Sum  Inputs=+-
  wires:
  Puck State/1 -> Data Store Write3/1
  Subtract/1 -> Custom Discrete PD (X-Position)/1(ex)
  Desired Py (BLUE)/1 -> Subtract1/1
  Custom Discrete PD (X-Position)/1(Fx) -> BLUE_Fx/1
  Desired Px (BLUE)/1 -> Subtract/1
  Subtract1/1 -> Custom Discrete PD (Y-Position)/1(ey)
  Hough Control/1(Err) -> Custom Discrete PD (Attitude)/1(ez)
  Desired Attitude (BLUE)/1 -> Hough Control/1(Ref)
  Custom Discrete PD (Attitude)/1(Tz) -> BLUE_Tz/1
  "BLUE_Py "/1 -> Subtract1/2
  Custom Discrete PD (Y-Position)/1(Fy) -> BLUE_Fy/1
  BLUE_Px/1 -> Subtract/2
  BLUE_Rz/1 -> Hough Control/2(Act)

== system BetaMacs/Phase #5: Hold Home/Change RED Behavior ==
  note: PD Control Law - RED
  note: Additional Blocks
  note: Additional blocks are stored above. Note that to control attitude using the RW, simply replace RED_Tz with RED_Tz_RW.
  note: A simple PD control law is used here to command the platform to it's initial position, as defined in the initializer.
  note: ARM Control Law - RED
  Action Port : ActionPort  ActionPortLabel=if(u1 == 1 | u2 == 1)
  Constant2 : Constant  Value=0
  Constant4 : Constant  Value=platformSelection
  Custom Discrete PD (Attitude) : Subsystem
  Custom Discrete PD (X-Position) : Subsystem
  Custom Discrete PD (Y-Position) : Subsystem
  Data Store Write3 : DataStoreWrite  DataStoreName=Float_State  IndexOptions=Index vector (dialog)  Indices=1  OutputSizes=1
  Desired Px (RED) : Constant  Value=home_states_RED(1)  SampleTime=-1
  Desired Py (RED) : Constant  Value=home_states_RED(2)  SampleTime=-1
  Desired Rz (RED) : Constant  Value=home_states_RED(3)  SampleTime=-1
  Hough Control : Subsystem
  If : If  IfExpression=u1 == 4 | u1 == 5 | u1 == 10 | u1 == 11  ShowElse=off
  Puck State : Constant
  RED+ARM : Subsystem  TreatAsAtomicUnit=on
  RED_Fx : DataStoreWrite  DataStoreName=RED_Fx  IndexOptions=Index vector (dialog)  Indices=1  OutputSizes=1
  RED_Fy : DataStoreWrite  DataStoreName=RED_Fy  IndexOptions=Index vector (dialog)  Indices=1  OutputSizes=1
  RED_Px : DataStoreRead  DataStoreName=RED_Px  IndexOptions=Index vector (dialog)  Indices=1  OutputSizes=1
  "RED_Py " : DataStoreRead  DataStoreName=RED_Py  IndexOptions=Index vector (dialog)  Indices=1  OutputSizes=1
  RED_Rz : DataStoreRead  DataStoreName=RED_Rz  IndexOptions=Index vector (dialog)  Indices=1  OutputSizes=1
  RED_Tz : DataStoreWrite  DataStoreName=RED_Tz  IndexOptions=Index vector (dialog)  Indices=1  OutputSizes=1
  RED_Tz_RW1 : DataStoreWrite  DataStoreName=RED_Tz_RW  IndexOptions=Index vector (dialog)  Indices=1  OutputSizes=1
  Subtract : Sum  Inputs=+-
  Subtract1 : Sum  Inputs=+-
  wires:
  Constant2/1 -> RED_Tz_RW1/1
  Desired Px (RED)/1 -> Subtract/1
  Custom Discrete PD (Attitude)/1(Tz) -> RED_Tz/1
  Desired Rz (RED)/1 -> Hough Control/1(Ref)
  RED_Rz/1 -> Hough Control/2(Act)
  Desired Py (RED)/1 -> Subtract1/1
  Custom Discrete PD (X-Position)/1(Fx) -> RED_Fx/1
  Subtract/1 -> Custom Discrete PD (X-Position)/1(ex)
  Hough Control/1(Err) -> Custom Discrete PD (Attitude)/1(ez)
  Custom Discrete PD (Y-Position)/1(Fy) -> RED_Fy/1
  RED_Px/1 -> Subtract/2
  "RED_Py "/1 -> Subtract1/2
  Subtract1/1 -> Custom Discrete PD (Y-Position)/1(ey)
  Puck State/1 -> Data Store Write3/1
  Constant4/1 -> If/1
  If/1 -> RED+ARM/Action

== system BetaMacs/Phase #6: Clean Shutdown/Change BLACK Behavior ==
  note: At the end of the experiment, the pucks must be turned off.
  note: At the end of the experiment, all thrust and arms movement must cease.
  Action Port : ActionPort  ActionPortLabel=if(u1 == 2 | u2 == 1)
  BLACK_Fx : DataStoreWrite  DataStoreName=BLACK_Fx  IndexOptions=Index vector (dialog)  Indices=1  OutputSizes=1
  BLACK_Fy : DataStoreWrite  DataStoreName=BLACK_Fy  IndexOptions=Index vector (dialog)  Indices=1  OutputSizes=1
  BLACK_Tz : DataStoreWrite  DataStoreName=BLACK_Tz  IndexOptions=Index vector (dialog)  Indices=1  OutputSizes=1
  Constant3 : Constant  Value=0
  Constant4 : Constant  Value=0
  Constant5 : Constant  Value=0
  Data Store Write3 : DataStoreWrite  DataStoreName=Float_State  IndexOptions=Index vector (dialog)  Indices=1  OutputSizes=1
  Puck State : Constant  Value=0
  wires:
  Constant3/1 -> BLACK_Fx/1
  Constant5/1 -> BLACK_Tz/1
  Constant4/1 -> BLACK_Fy/1
  Puck State/1 -> Data Store Write3/1

== system BetaMacs/Phase #6: Clean Shutdown/Change BLUE Behavior ==
  note: Before getting good data, the platforms must NOT be floating. So, float is set to be "off".
  note: For the initialization phase, we do not want any thrust. Thus, all commanded forces are zero.
  Action Port : ActionPort  ActionPortLabel=if(u1 == 3 | u2 == 1)
  BLUE_Fx : DataStoreWrite  DataStoreName=BLUE_Fx  IndexOptions=Index vector (dialog)  Indices=1  OutputSizes=1
  BLUE_Fy : DataStoreWrite  DataStoreName=BLUE_Fy  IndexOptions=Index vector (dialog)  Indices=1  OutputSizes=1
  BLUE_Tz : DataStoreWrite  DataStoreName=BLUE_Tz  IndexOptions=Index vector (dialog)  Indices=1  OutputSizes=1
  Constant3 : Constant  Value=0
  Constant4 : Constant  Value=0
  Constant5 : Constant  Value=0
  Data Store Write4 : DataStoreWrite  DataStoreName=Float_State  IndexOptions=Index vector (dialog)  Indices=1  OutputSizes=1
  Puck State : Constant  Value=0
  wires:
  Constant3/1 -> BLUE_Fx/1
  Constant5/1 -> BLUE_Tz/1
  Constant4/1 -> BLUE_Fy/1
  Puck State/1 -> Data Store Write4/1

== system BetaMacs/Phase #6: Clean Shutdown/Change RED Behavior ==
  note: At the end of the experiment, the pucks must be turned off.
  note: At the end of the experiment, all thrust and arms movement must cease.
  note: Once the platform has settled, the RW must be slowly desaturated (assuming it has been used).
  Action Port : ActionPort  ActionPortLabel=if(u1 == 1 | u2 == 1)
  Constant{,1..3} (4 alike) : Constant  Value=0
  Data Store Write1 : DataStoreWrite  DataStoreName=RED_ARM_Control_Mode  IndexOptions=Index vector (dialog)  Indices=1  OutputSizes=1
  Data Store Write3 : DataStoreWrite  DataStoreName=Float_State  IndexOptions=Index vector (dialog)  Indices=1  OutputSizes=1
  Gain : Gain  Gain=-1
  Puck State : Constant  Value=0
  RED_Fx : DataStoreWrite  DataStoreName=RED_Fx  IndexOptions=Index vector (dialog)  Indices=1  OutputSizes=1
  RED_Fy : DataStoreWrite  DataStoreName=RED_Fy  IndexOptions=Index vector (dialog)  Indices=1  OutputSizes=1
  RED_Tz : DataStoreWrite  DataStoreName=RED_Tz  IndexOptions=Index vector (dialog)  Indices=1  OutputSizes=1
  RED_Tz_RW : DataStoreWrite  DataStoreName=RED_Tz_RW  IndexOptions=Index vector (dialog)  Indices=1  OutputSizes=1
  RED_dRz_Speed : DataStoreRead  DataStoreName=RED_dRz_RW_Sat  IndexOptions=Index vector (dialog)  Indices=1  OutputSizes=1
  Saturation : Saturate  UpperLimit=0.005  LowerLimit=-0.005
  wires:
  Constant/1 -> RED_Fx/1
  RED_dRz_Speed/1 -> Gain/1
  Saturation/1 -> RED_Tz_RW/1
  Constant1/1 -> RED_Fy/1
  Gain/1 -> Saturation/1
  Constant2/1 -> RED_Tz/1
  Puck State/1 -> Data Store Write3/1
  Constant3/1 -> Data Store Write1/1

== system BetaMacs/PhaseSpace Camera Code/Initialize Universal Time (Simulation) ==
  Action Port : ActionPort  ActionPortLabel=elseif(u1 == 1)
  Set Universal Time (If this is a simulation) : Clock
  Universal_Time : DataStoreWrite  DataStoreName=Univ_Time  IndexOptions=Index vector (dialog)  Indices=1  OutputSizes=1
  wires:
  Set Universal Time (If this is a simulation)/1 -> Universal_Time/1
